simulink model "pfb_fir_128c_2p_16i_8b_core"  (R2019a)
settings: Solver=ode45  StartTime=0.0  StopTime=10.0  RelTol=1e-3  EnableMultiTasking=on
undefined symbols (not defined in the file or in its folder): pfb_coeff_gen_calc
libraries: xbsIndex_r4 x2538, casper_library_delays x224, casper_library_misc x176, simulink x3
(part 1 of 29)
settings Model: Creator=zaki  LastModifiedBy=jackh
settings DataIOCC: LimitDataPoints=on  SaveFormat=Array  SignalLoggingSaveFormat=ModelDataLogs  ReturnWorkspaceOutputs=off
settings OptimizationCC: ExpressionDepthLimit=2147483647  LifeSpan=inf
settings DebuggingCC: UnderspecifiedInitializationDetection=Classic  MergeDetectMultiDrivingBlocksExec=none  SolverPrmCheckMsg=warning  FcnCallInpInsideContextMsg=warning  StateNameClashWarn=warning  SFUnexpectedBacktrackingDiag=warning  SFNoUnconditionalDefaultTransitionDiag=warning  SFExecutionAtInitializationDiag=none  ArithmeticOperatorsInVariantConditions=warning
settings HardwareCC: ProdBitPerPointer=32  ProdBitPerSizeT=32  ProdBitPerPtrDiffT=32  ProdLargestAtomicFloat=None  ProdIntDivRoundTo=Undefined  ProdEndianess=Unspecified  ProdWordSize=32  ProdHWDeviceType=32-bit Generic
settings ModelReferenceCC: PropagateSignalLabelsOutOfModel=off
settings SFSimCC: SimUseLocalCustomCode=off
settings RTWCC: RTWUseLocalCustomCode=off
settings CodeAppCC: StateflowObjectComments=on
settings GRTTargetCC: TargetLangStandard=C89/C90 (ANSI)  GeneratePreprocessorConditionals=Disable all  CombineOutputUpdateFcns=off  GRTInterface=on
settings ConfigComp: CovMetricSettings=dw  CovHtmlReporting=on  CovSaveCumulativeToWorkspaceVar=on  CovSaveSingleToWorkspaceVar=on  CovExternalEMLEnable=off

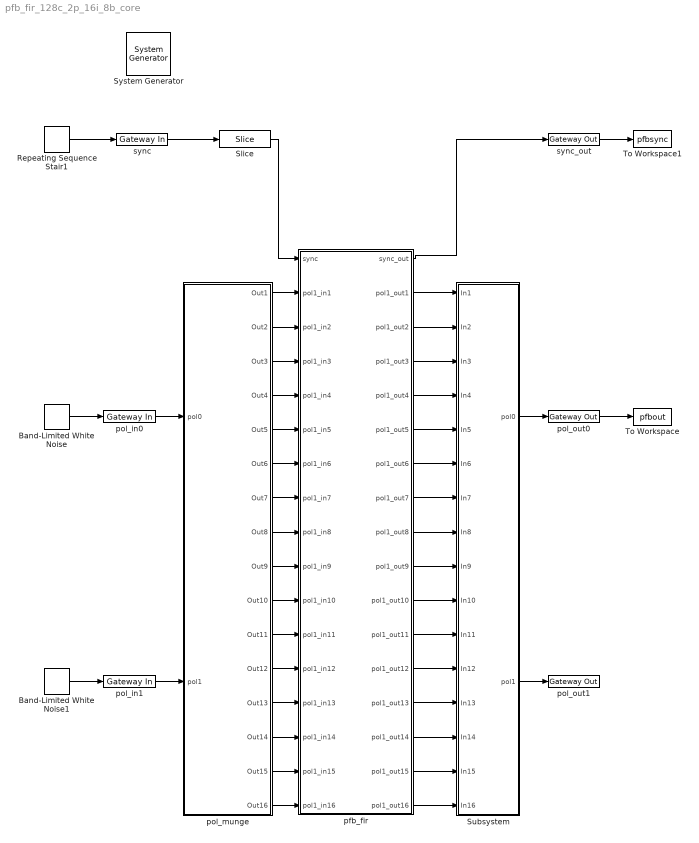
== system pfb_fir_128c_2p_16i_8b_core ==
  " System Generator" : xbsIndex_r4/ System Generator  Tag=genX  xilinxfamily=virtexuplusHBM  part=xcvu37p  speed=-2-e  package=fsvh2892  synthesis_tool=Synplify Pro  clock_wrapper=Clock Enables  directory=./pfb_fir_128c_2p_16i_8b_core  proj_type=Project Navigator  Synth_file=XST Defaults  Impl_file=ISE Defaults  testbench=off  simulink_period=1  sysclk_period=5  dcm_input_clock_period=100  incr_netlist=off  trim_vbits=Everywhere in SubSystem  dbl_ovrd=According to Block Masks  core_generation=According to Block Masks  run_coregen=off  deprecated_control=off  eval_field=0  block_type=sysgen
      settings: block_version=10.1.3
  Band-Limited White Noise : simulink/Sources/Band-Limited White Noise  Cov=(16/128)^2  Ts=1  seed=[23341]
  Band-Limited White Noise1 : simulink/Sources/Band-Limited White Noise  Cov=(16/128)^2  Ts=1  seed=[23341]
  Repeating Sequence Stair1 : simulink/Sources/Repeating Sequence Stair  OutValues=[1, zeros(1,2^12-1)]  tsamp=1  OutMin=[]  OutMax=[]  OutDataTypeStr=float('double')  OutputDataTypeScalingMode=Specify via dialog  OutDataType=float('double')  ConRadixGroup=Best Precision: Vector-wise  OutScaling=2^-12
  Slice : xbsIndex_r4/Slice  nbits=3  boolean_output=on  mode=Lower Bit Location + Width  bit1=0  base1=MSB of Input  bit0=0  base0=LSB of Input  dbl_ovrd=off  block_type=slice
  Subsystem : Subsystem
  To Workspace : ToWorkspace  VariableName=pfbout  SampleTime=-1
  To Workspace1 : ToWorkspace  VariableName=pfbsync  SampleTime=-1
  pfb_fir : Subsystem  Tag=casper:pfb_fir  AncestorBlock=casper_library_pfbs/pfb_fir  mask(pfb_fir){PFBSize=8, TotalTaps=8, WindowType=hamming, n_inputs=4, MakeBiplex=off, BitWidthIn=8, BitWidthOut=18, CoeffBitWidth=18, CoeffDistMem=off, add_latency=1, mult_latency=2, bram_latency=2, fan_latency=1, quantization=Round  (unbiased: Even Values), fwidth=1, mult_spec=2, coeffs_share=on}
      mask prompts: PFBSize "Size of PFB: (2^? pnts)"; TotalTaps "Total Number of Taps:"; WindowType "Windowing Function:"; n_inputs "Number of Simultaneous Inputs: (2^?)"; MakeBiplex "Make Biplex?"; BitWidthIn "Input Bitwidth:"; BitWidthOut "Output Bitwidth:"; CoeffBitWidth "Coefficient Bitwidth:"; CoeffDistMem "Use Distributed Memory for Coeffs"; add_latency "Add Latency"; mult_latency "Mult Latency"; bram_latency "BRAM Latency"; fan_latency "Fanout Latency"; quantization "Quantization Behavior"; fwidth "Bin Width Scaling (normal=1)"; mult_spec "Multiplier specification (0=core, 1=embedded, 2=behavioural) (left=1st tap, or just one value)"; coeffs_share "Share coefficients between polarisations (use less BRAM)?"
      mask init:
      | pfb_fir_init(gcb, ...
      |     'PFBSize', PFBSize, ...
      |     'TotalTaps', TotalTaps, ...
      |     'WindowType', WindowType, ...
      |     'n_inputs', n_inputs, ...
      |     'MakeBiplex', MakeBiplex, ...
      |     'BitWidthIn', BitWidthIn, ...
      |     'BitWidthOut', BitWidthOut, ...
      |     'CoeffBitWidth', CoeffBitWidth, ...
      |     'CoeffDistMem', CoeffDistMem, ...
      |     'add_latency', add_latency, ...
      |     'mult_latency', mult_latency, ...
      |     'bram_latency', bram_latency, ...
      |     'fan_latency', fan_latency, ...
      |     'quantization', quantization, ...
      |     'fwidth', fwidth, ...
      |     'mult_spec', mult_spec, ...
      |     'coeffs_share', coeffs_share);
      settings: AttributesFormatString=|
      | taps=8, add_latency=1
      | max scale 0.823
      mask Help: eval('xlWeb(''http://casper.berkeley.edu/wiki/Pfb_fir'')')
      mask Callback TotalTaps:
      | %num_taps = eval(get_param(gcb, 'TotalTaps'));
      | %old_vec = eval(get_param(gcb, 'mult_spec'));
      | 
      | %vec = 2.*ones(1,num_taps);
      | %old_size = length(old_vec);
      | 
      | %if(old_size <= num_taps),
      | %   new_size = old_size;
      | %else,
      | %    new_size = num_taps;
      | %end
      | 
      | %for n = 1:new_size, vec(n) = old_vec(n); end
      | %set_param(gcb, 'mult_spec', mat2str(vec));
      mask TypeOptions WindowType: bartlett | barthannwin | blackman | blackmanharris | bohamwin | chebwin | flattopwin | gausswin | hamming | hann | kaiser | nuttallwin | parzenwin | rectwin | tukeywin | triang | userwindow
      mask TypeOptions quantization: Truncate | Round  (unbiased: +/- Inf) | Round  (unbiased: Even Values)
      mask Callback fwidth:
      | %num_taps = eval(get_param(gcb, 'TotalTaps'));
      | %old_vec = eval(get_param(gcb, 'mult_spec'));
      | 
      | %vec = 2.*ones(1,num_taps);
      | %old_size = length(old_vec);
      | 
      | %if(old_size <= num_taps),
      | %    new_size = old_size;
      | %else,
      | %    new_size = num_taps;
      | %end
      | 
      | %for n = 1:new_size, vec(n) = old_vec(n); end
      | %set_param(gcb, 'mult_spec', mat2str(vec));
      mask Callback mult_spec:
      | %num_taps = eval(get_param(gcb, 'TotalTaps'));
      | %old_vec = eval(get_param(gcb, 'mult_spec'));
      | 
      | %vec = 2.*ones(1,num_taps);
      | %old_size = length(old_vec);
      | 
      | %if(old_size <= num_taps),
      | %    new_size = old_size;
      | %else,
      | %    new_size = num_taps;
      | %end
      | 
      | %for n = 1:new_size, vec(n) = old_vec(n); end
      | %set_param(gcb, 'mult_spec', mat2str(vec));
  pol_in0 : xbsIndex_r4/Gateway In  gui_display_data_type=Fixed-point  arith_type=Unsigned  n_bits=8*16  bin_pt=0  preci_type=Single  exp_width=8  frac_width=24  rows=1  columns=1  quantization="Round  (unbiased: +/- Inf)"  overflow=Saturate  period=1  UseAsADC=off  ADCChannel='1'  interface=None  automatic_assignment=on  address_offset=hex2dec('00')  intf_name=''  intf_description=''  default_value=0  timing_constraint=None  locs_specified=off  LOCs={}  io_standard={}  inherit_from_input=off  hdl_port=on  dbl_ovrd=off  block_type=gatewayin
      settings: block_version=10.1.3
  pol_in1 : xbsIndex_r4/Gateway In  gui_display_data_type=Fixed-point  arith_type=Unsigned  n_bits=8*16  bin_pt=0  preci_type=Single  exp_width=8  frac_width=24  rows=1  columns=1  quantization="Round  (unbiased: +/- Inf)"  overflow=Saturate  period=1  UseAsADC=off  ADCChannel='1'  interface=None  automatic_assignment=on  address_offset=hex2dec('00')  intf_name=''  intf_description=''  default_value=0  timing_constraint=None  locs_specified=off  LOCs={}  io_standard={}  inherit_from_input=off  hdl_port=on  dbl_ovrd=off  block_type=gatewayin
      settings: block_version=10.1.3
  pol_munge : Subsystem
  pol_out0 : xbsIndex_r4/Gateway Out  inherit_from_input=off  hdl_port=on  rows=1  columns=1  UseAsDAC=off  DACChannel='1'  interface=None  automatic_assignment=on  address_offset=hex2dec('00')  intf_name=''  intf_description=''  timing_constraint=None  locs_specified=off  LOCs={}  io_standard={}  block_type=gatewayout
      settings: infoedit="Gateway out block.  Converts Xilinx fixed point inputs into ouputs of type Simulink integer, double, or fixed point.<P><P>Hardware notes:  In hardware these blocks become top level output ports or are discarded, depending on how they are configured."  block_version=10.1.3
  pol_out1 : xbsIndex_r4/Gateway Out  inherit_from_input=off  hdl_port=on  rows=1  columns=1  UseAsDAC=off  DACChannel='1'  interface=None  automatic_assignment=on  address_offset=hex2dec('00')  intf_name=''  intf_description=''  timing_constraint=None  locs_specified=off  LOCs={}  io_standard={}  block_type=gatewayout
      settings: infoedit="Gateway out block.  Converts Xilinx fixed point inputs into ouputs of type Simulink integer, double, or fixed point.<P><P>Hardware notes:  In hardware these blocks become top level output ports or are discarded, depending on how they are configured."  block_version=10.1.3
  sync : xbsIndex_r4/Gateway In  gui_display_data_type=Fixed-point  arith_type=Unsigned  n_bits=32  bin_pt=0  preci_type=Single  exp_width=8  frac_width=24  rows=1  columns=1  quantization="Round  (unbiased: +/- Inf)"  overflow=Saturate  period=1  UseAsADC=off  ADCChannel='1'  interface=None  automatic_assignment=on  address_offset=hex2dec('00')  intf_name=''  intf_description=''  default_value=0  timing_constraint=None  locs_specified=off  LOCs={}  io_standard={}  inherit_from_input=off  hdl_port=on  dbl_ovrd=off  block_type=gatewayin
      settings: block_version=10.1.3
  sync_out : xbsIndex_r4/Gateway Out  inherit_from_input=off  hdl_port=on  rows=1  columns=1  UseAsDAC=off  DACChannel='1'  interface=None  automatic_assignment=on  address_offset=hex2dec('00')  intf_name=''  intf_description=''  timing_constraint=None  locs_specified=off  LOCs={}  io_standard={}  block_type=gatewayout
      settings: infoedit="Gateway out block.  Converts Xilinx fixed point inputs into ouputs of type Simulink integer, double, or fixed point.<P><P>Hardware notes:  In hardware these blocks become top level output ports or are discarded, depending on how they are configured."  block_version=10.1.3
  wires:
  sync/1 -> Slice/1
  Band-Limited White Noise/1 -> pol_in0/1
  pol_out0/1 -> To Workspace/1
  Repeating Sequence Stair1/1 -> sync/1
  sync_out/1 -> To Workspace1/1
  pfb_fir/1(sync_out) -> sync_out/1
  Slice/1 -> pfb_fir/1(sync)
  pol_munge/1(Out1) -> pfb_fir/2(pol1_in1)
  pol_munge/2(Out2) -> pfb_fir/3(pol1_in2)
  pol_munge/3(Out3) -> pfb_fir/4(pol1_in3)
  pol_munge/4(Out4) -> pfb_fir/5(pol1_in4)
  pol_munge/5(Out5) -> pfb_fir/6(pol1_in5)
  pol_munge/6(Out6) -> pfb_fir/7(pol1_in6)
  pol_munge/7(Out7) -> pfb_fir/8(pol1_in7)
  pol_munge/8(Out8) -> pfb_fir/9(pol1_in8)
  pol_munge/9(Out9) -> pfb_fir/10(pol1_in9)
  pol_munge/10(Out10) -> pfb_fir/11(pol1_in10)
  pol_munge/11(Out11) -> pfb_fir/12(pol1_in11)
  pol_munge/12(Out12) -> pfb_fir/13(pol1_in12)
  pol_munge/13(Out13) -> pfb_fir/14(pol1_in13)
  pol_munge/14(Out14) -> pfb_fir/15(pol1_in14)
  pol_munge/15(Out15) -> pfb_fir/16(pol1_in15)
  pol_munge/16(Out16) -> pfb_fir/17(pol1_in16)
  pol_in0/1 -> pol_munge/1(pol0)
  Band-Limited White Noise1/1 -> pol_in1/1
  pol_in1/1 -> pol_munge/2(pol1)
  pfb_fir/2(pol1_out1) -> Subsystem/1(In1)
  pfb_fir/3(pol1_out2) -> Subsystem/2(In2)
  pfb_fir/4(pol1_out3) -> Subsystem/3(In3)
  pfb_fir/5(pol1_out4) -> Subsystem/4(In4)
  pfb_fir/6(pol1_out5) -> Subsystem/5(In5)
  pfb_fir/7(pol1_out6) -> Subsystem/6(In6)
  pfb_fir/8(pol1_out7) -> Subsystem/7(In7)
  pfb_fir/9(pol1_out8) -> Subsystem/8(In8)
  pfb_fir/10(pol1_out9) -> Subsystem/9(In9)
  pfb_fir/11(pol1_out10) -> Subsystem/10(In10)
  pfb_fir/12(pol1_out11) -> Subsystem/11(In11)
  pfb_fir/13(pol1_out12) -> Subsystem/12(In12)
  pfb_fir/14(pol1_out13) -> Subsystem/13(In13)
  pfb_fir/15(pol1_out14) -> Subsystem/14(In14)
  pfb_fir/16(pol1_out15) -> Subsystem/15(In15)
  pfb_fir/17(pol1_out16) -> Subsystem/16(In16)
  Subsystem/1(pol0) -> pol_out0/1
  Subsystem/2(pol1) -> pol_out1/1

== system pfb_fir_128c_2p_16i_8b_core/Subsystem ==
  In1 : Inport
  In2 : Inport  Port=2
  In3 : Inport  Port=3
  In4 : Inport  Port=4
  In5 : Inport  Port=5
  In6 : Inport  Port=6
  In7 : Inport  Port=7
  In8 : Inport  Port=8
  In9 : Inport  Port=9
  In10 : Inport  Port=10
  In11 : Inport  Port=11
  In12 : Inport  Port=12
  In13 : Inport  Port=13
  In14 : Inport  Port=14
  In15 : Inport  Port=15
  In16 : Inport  Port=16
  bus_create1 : Subsystem  AncestorBlock=casper_library_flow_control/bus_create  mask(bus_create){inputNum=16}
      mask prompts: inputNum "Number of inputs:"
      mask init:
      | bus_create_init(gcb,...
      |     'inputNum', inputNum);
  bus_create2 : Subsystem  AncestorBlock=casper_library_flow_control/bus_create  mask(bus_create){inputNum=16}
      mask prompts: inputNum "Number of inputs:"
      mask init:
      | bus_create_init(gcb,...
      |     'inputNum', inputNum);
  c_to_ri{,1..15} (16 alike) : casper_library_misc/c_to_ri  n_bits=18  bin_pt=17
      settings: SourceProductName=CASPER DSP Blockset
  pol0 : Outport
  pol1 : Outport  Port=2
  wires:
  In16/1 -> c_to_ri15/1
  c_to_ri5/2 -> bus_create2/6(in6)
  c_to_ri14/1 -> bus_create1/15(in15)
  c_to_ri11/1 -> bus_create1/12(in12)
  c_to_ri4/2 -> bus_create2/5(in5)
  c_to_ri13/2 -> bus_create2/14(in14)
  c_to_ri14/2 -> bus_create2/15(in15)
  c_to_ri9/1 -> bus_create1/10(in10)
  c_to_ri8/2 -> bus_create2/9(in9)
  c_to_ri9/2 -> bus_create2/10(in10)
  In9/1 -> c_to_ri8/1
  In4/1 -> c_to_ri3/1
  In8/1 -> c_to_ri7/1
  c_to_ri3/2 -> bus_create2/4(in4)
  In3/1 -> c_to_ri2/1
  c_to_ri1/1 -> bus_create1/2(in2)
  c_to_ri10/2 -> bus_create2/11(in11)
  In10/1 -> c_to_ri9/1
  In13/1 -> c_to_ri12/1
  In7/1 -> c_to_ri6/1
  c_to_ri7/2 -> bus_create2/8(in8)
  c_to_ri12/1 -> bus_create1/13(in13)
  c_to_ri11/2 -> bus_create2/12(in12)
  c_to_ri15/1 -> bus_create1/16(in16)
  In15/1 -> c_to_ri14/1
  In1/1 -> c_to_ri/1
  c_to_ri13/1 -> bus_create1/14(in14)
  c_to_ri/2 -> bus_create2/1(in1)
  c_to_ri6/1 -> bus_create1/7(in7)
  c_to_ri4/1 -> bus_create1/5(in5)
  c_to_ri12/2 -> bus_create2/13(in13)
  c_to_ri7/1 -> bus_create1/8(in8)
  In14/1 -> c_to_ri13/1
  c_to_ri6/2 -> bus_create2/7(in7)
  In12/1 -> c_to_ri11/1
  In5/1 -> c_to_ri4/1
  c_to_ri2/2 -> bus_create2/3(in3)
  c_to_ri1/2 -> bus_create2/2(in2)
  In2/1 -> c_to_ri1/1
  c_to_ri15/2 -> bus_create2/16(in16)
  c_to_ri10/1 -> bus_create1/11(in11)
  bus_create2/1(bus_out) -> pol1/1
  c_to_ri/1 -> bus_create1/1(in1)
  c_to_ri8/1 -> bus_create1/9(in9)
  c_to_ri3/1 -> bus_create1/4(in4)
  c_to_ri5/1 -> bus_create1/6(in6)
  In11/1 -> c_to_ri10/1
  bus_create1/1(bus_out) -> pol0/1
  In6/1 -> c_to_ri5/1
  c_to_ri2/1 -> bus_create1/3(in3)
